simulink model "wes268a_prelab1"  (R2015b)
settings: Solver=VariableStepAuto  StartTime=0.0  StopTime=1536  RelTol=1e-3
libraries: dspsrcs4 x2, dspsigops x1
settings Model: Creator=jemele  LastModifiedBy=jemele

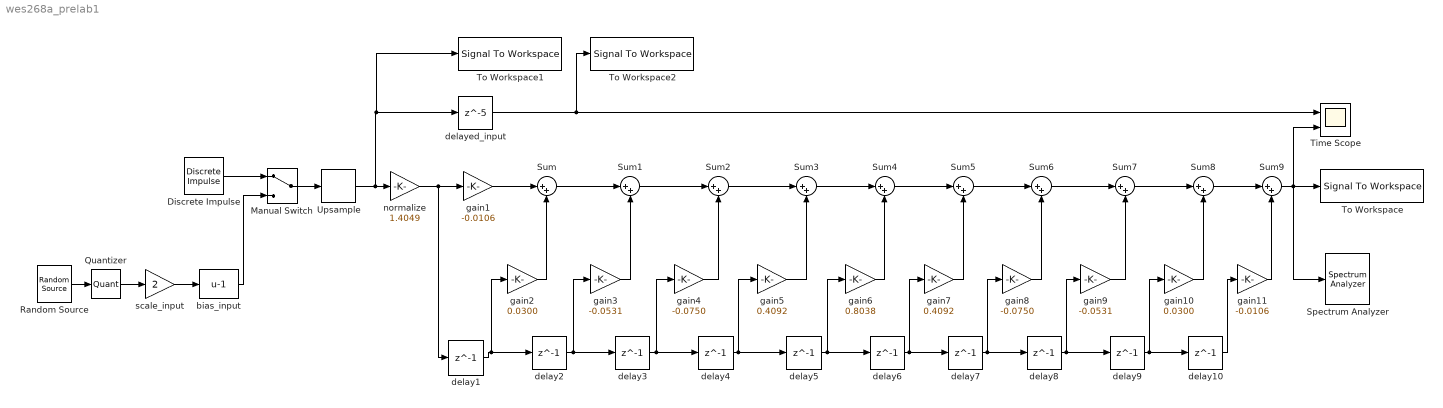
== system wes268a_prelab1 ==
  Discrete Impulse : dspsrcs4/Discrete  Impulse  Delay=0  SampleTime=1  FrameSample=1536  OutputFrames=off  dataType=double  isSigned=on  wordLen=16  udDataType=sfix(16)  fracBitsMode=Best precision  numFracBits=15  OutDataTypeStr=double  LastOutDataTypeStr=double
  Manual Switch : ManualSwitch
  Quantizer : Quantizer  QuantizationInterval=1
  Random Source : dspsrcs4/Random Source  SrcType=Uniform  NormMethod=Ziggurat  CltLength=12  MinVal=0  MaxVal=1  MeanVal=0  VarVal=1  RepMode=Not repeatable  rawSeed=1  IsInherit=off  SampMode=Discrete  SampTime=1  SampFrame=1  DataType=Double  OutComplex=Real  OutputFrames=off
  Spectrum Analyzer : SpectrumAnalyzer
  Sum{,1..9} (10 alike) : Sum  Inputs=|++
  Time Scope : Scope  NumInputPorts=2
  To Workspace : SignalToWorkspace  VariableName=sim_output
  To Workspace1 : SignalToWorkspace  VariableName=sim_input
  To Workspace2 : SignalToWorkspace  VariableName=sim_delayed_input
  Upsample : dspsigops/Upsample  N=2  phase=0  InputProcessing=Columns as channels (frame based)  RateOptions=Allow multirate processing  ic=0  mode=Unused parameter value
  bias_input : Bias  Bias=-1
  delay{1..10} (10 alike) : Delay  DelayLength=1
  delayed_input : Delay  DelayLength=5
  gain1 : Gain  Gain=-0.0106
  gain10 : Gain  Gain=0.0300
  gain11 : Gain  Gain=-0.0106
  gain2 : Gain  Gain=0.0300
  gain3 : Gain  Gain=-0.0531
  gain4 : Gain  Gain=-0.0750
  gain5 : Gain  Gain=0.4092
  gain6 : Gain  Gain=0.8038
  gain7 : Gain  Gain=0.4092
  gain8 : Gain  Gain=-0.0750
  gain9 : Gain  Gain=-0.0531
  normalize : Gain  Gain=1.4049
  scale_input : Gain  Gain=2
  wires:
  Sum/1 -> Sum1/1
  gain1/1 -> Sum/1
  gain2/1 -> Sum/2
  delay1/1 -> gain2/1, delay2/1
  gain3/1 -> Sum1/2
  delay2/1 -> delay3/1, gain3/1
  delay3/1 -> delay4/1, gain4/1
  delay4/1 -> delay5/1, gain5/1
  gain4/1 -> Sum2/2
  Sum1/1 -> Sum2/1
  delay5/1 -> delay6/1, gain6/1
  gain5/1 -> Sum3/2
  Sum2/1 -> Sum3/1
  gain6/1 -> Sum4/2
  Sum3/1 -> Sum4/1
  delay6/1 -> gain7/1, delay7/1
  delay7/1 -> delay8/1, gain8/1
  delay8/1 -> gain9/1, delay9/1
  delay9/1 -> delay10/1, gain10/1
  gain7/1 -> Sum5/2
  Sum4/1 -> Sum5/1
  gain8/1 -> Sum6/2
  Sum5/1 -> Sum6/1
  gain9/1 -> Sum7/2
  Sum6/1 -> Sum7/1
  gain10/1 -> Sum8/2
  Sum7/1 -> Sum8/1
  delay10/1 -> gain11/1
  gain11/1 -> Sum9/2
  Sum8/1 -> Sum9/1
  Discrete Impulse/1 -> Manual Switch/1
  Random Source/1 -> Quantizer/1
  Quantizer/1 -> scale_input/1
  scale_input/1 -> bias_input/1
  bias_input/1 -> Manual Switch/2
  Sum9/1 -> Spectrum Analyzer/1, Time Scope/2, To Workspace/1
  delayed_input/1 -> To Workspace2/1, Time Scope/1
  Manual Switch/1 -> Upsample/1
  normalize/1 -> gain1/1, delay1/1
  Upsample/1 -> To Workspace1/1, delayed_input/1, normalize/1
